simulink model "warmup3"  (R2018b)
settings: Solver=VariableStepAuto  StartTime=0.0  StopTime=10.0  RelTol=1e-3
libraries: audiosources x1, dspsnks4 x1
settings Model: Creator=Jason  LastModifiedBy=Jason
settings SFSimCC: SimUseLocalCustomCode=off
settings RTWCC: RTWUseLocalCustomCode=off
settings CodeAppCC: StateflowObjectComments=on

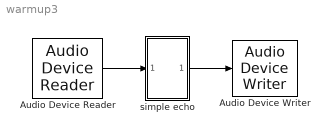
== system warmup3 ==
  Audio Device Reader : audiosources/Audio Device Reader  Driver=DirectSound  Device=Default  SampleRate=44100  NumChannels=1  SamplesPerFrame=1024  BitDepth=16-bit integer  NumBuffers=10  DefaultInputChannelMapping=on  InputChannelMapping=1:2  OutputNumOverrunSamples=off  OutputDataType=double  DriverIdx=1  DeviceWarnFlag=''
      settings: SourceProductName=Audio System Toolbox  SourceProductBaseCode=AU
  Audio Device Writer : dspsnks4/Audio Device Writer  Driver=DirectSound  Device=Default  InheritSampleRate=off  SampleRate=44100  BitDepth=16-bit integer  BufferSize=4096  NumBuffers=10  DefaultOutputChannelMapping=on  OutputChannelMapping=1:2  OutputNumUnderrunSamples=off  DriverIdx=1  DeviceWarnFlag=''
  "simple echo " : Subsystem
  wires:
  Audio Device Reader/1 -> "simple echo "/1(In1)
  "simple echo "/1(Out1) -> Audio Device Writer/1

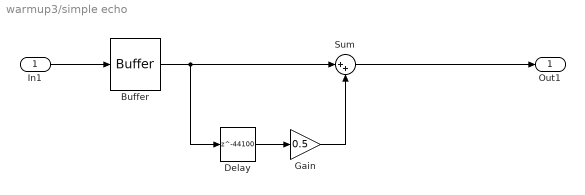
== system warmup3/simple echo  ==
  In1 : Inport
  Buffer : Buffer  N=128  OutputFrames=off
  Delay : Delay  DelayLength=44100  InitialCondition=0  InputProcessing=Columns as channels (frame based)
  Gain : Gain  Gain=0.5
  Sum : Sum  Inputs=|++
  Out1 : Outport
  wires:
  Delay/1 -> Gain/1
  Buffer/1 -> Delay/1, Sum/1
  Gain/1 -> Sum/2
  In1/1 -> Buffer/1
  Sum/1 -> Out1/1
